simulink model "sensorFusionWithControlTB66"  (R2024a)
settings: Solver=FixedStepAuto  StartTime=0.0  StopTime=inf  FixedStep=controlRate  RelTol=1e-3
InitFcn:
  | modelParamsDD = Simulink.data.dictionary.open('modelConfigData.sldd');
  | sectModel = getSection(modelParamsDD,'Design Data');
  | controlRateTemp = getValue(getEntry(sectModel,'controlRate'));
  | 
  | measRate = controlRateTemp;
  | angleEstRate = measRate;
  | stateEstRate = measRate;
  | 
  | % Complementary filter
  | fc = 5; %Hz
  | tau = 1/(2*pi*fc);
  | % alpha = tau/(tau+controlRateTemp);
  | alpha = 0.98;
  | 
  | % Control params
  | tiltSetPoint = 5; % degree
  | D_min = 0;
  | 
  | % Tilt angle PID
  | Tw = 1;
  | Kp = 28;
  | Ki = 10; % At 100 Hz
  | Kd = 0;
  | 
  | 
  | clear controlRateTemp
undefined symbols (not defined in the file or in its folder): accelToUnit, controlRate, gyroToUnit, MaxMotorVoltage
libraries: stm32f7xxblockslib x2, stm32f4xxblockslib x1
settings Model: DataDictionary=globalData.sldd  VariantConfigurationObject=RobotVariantConfig  STM32="{\"PWMOutput\":[{\"ID\":\"sensorFusionWithControlTB66:205\"},{\"ID\":\"sensorFusionWithControlTB66:189\"}],\"DigitalPortWrite\":[{\"ID\":\"sensorFusionWithControlTB66:1189\"},{\"ID\":\"sensorFusionWithControlTB66:1220\"},{\"ID\":\"sensorFusionWithControlTB66:1221\"},{\"ID\":\"sensorFusionWithControlTB66:1222\"},{\"ID\":\"sensorFusionWithControlTB66:1223\"},{\"ID\":\"sensorFusionWithControlTB66:1225:7\"},{\"ID\":\"sensorFusionWithControlTB66:1225:8\"},{\"ID\":\"sensorFusionWithControlTB66:1225:9\"},{\"ID\":\"sensorFusionWithControlTB66:1225:10\"}],\"I2CControllerRead\":[{\"ID\":\"sensorFusionWithControlTB66:1237:7\"},{\"ID\":\"sensorFusionWithControlTB66:1237:18\"},{\"ID\":\"sensorFusionWithControlTB66:1237:19\"},{\"ID\":\"sensorFusionWithControlTB66:1237:20\"},{\"ID\":\"sensorFusionWithControlTB66:1238:7\"},{\"ID\":\"sensorFusionWithControlTB66:1238:15\"},{\"ID\":\"sensorFusionWithControlTB66:1238:16\"},{\"ID\":\"sensorFusionWithControlTB66:1238:17\"}],\"I2CControllerWrite\":[{\"ID\":\"sensorFusionWithControlTB66:1237:21\"},{\"ID\":\"sensorFusionWithControlTB66:1237:22\"},{\"ID\":\"sensorFusionWithControlTB66:1237:23\"},{\"ID\":\"sensorFusionWithControlTB66:1238:18\"},{\"ID\":\"sensorFusionWithControlTB66:1238:19\"},{\"ID\":\"sensorFusionWithControlTB66:1238:20\"}]}"  SimulationMode=external  Creator=Peter  LastModifiedBy=Peter
settings OptimizationCC: OptimizeBlockIOStorage=off  BufferReuse=off  ReuseModelBlockBuffer=off  GlobalBufferReuse=off  ExpressionFolding=off  EnableMemcpy=off  PassReuseOutputArgsAs=Individual arguments  LocalBlockOutputs=off  ZeroExternalMemoryAtStartup=off  ZeroInternalMemoryAtStartup=off  MaxStackSize=64  OptimizeDataStoreBuffers=off  BusAssignmentInplaceUpdate=off  OptimizationLevel=level0  OptimizationCustomize=off  EfficientTunableParamExpr=on
settings DebuggingCC: ParameterTunabilityLossMsg=error
settings HardwareCC: ProdBitPerPointer=32  ProdBitPerSizeT=32  ProdBitPerPtrDiffT=32  ProdLargestAtomicInteger=Long  ProdLargestAtomicFloat=Double  ProdWordSize=32  ProdLongLongMode=on  ProdHWDeviceType=ARM Compatible->ARM Cortex-M
settings SFSimCC: MATLABDynamicMemAlloc=off
settings RTWCC: Description=Embedded Coder  SystemTargetFile=ert.tlc  HardwareBoard=STM32F7xx Based (Single precision FPU)  TemplateMakefile=ert_default_tmf  Toolchain=GNU Tools for ARM Embedded Processors
settings CodeAppCC: GenerateComments=off  IgnoreCustomStorageClasses=off  OperatorAnnotations=on  SimulinkDataObjDesc=on  SFDataObjDesc=on  SimulinkBlockComments=off
settings ERTTargetCC: TargetLangStandard=C99 (ISO)  CodeReplacementLibrary=ARM Cortex-M  SupportComplex=off  ExtMode=on  ExtModeTransport=3  ExtModeStaticAlloc=on  ExtModeStaticAllocSize=2048  ExtModeMexFile=ext_xcp  ExtModeMexArgs=1 'COM11' 115200  ExtModeIntrfLevel=Level2 - Open

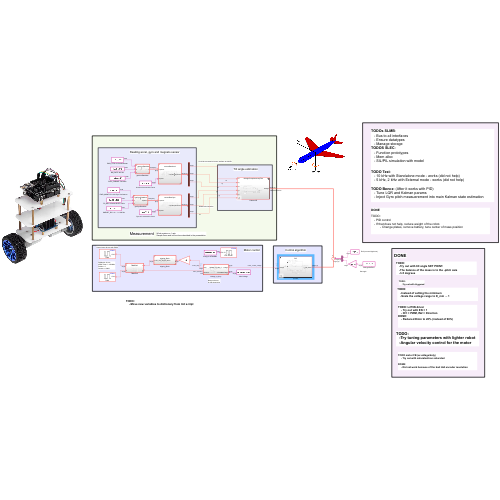
[thumbnail: Simulink's stored preview of the top-level diagram]
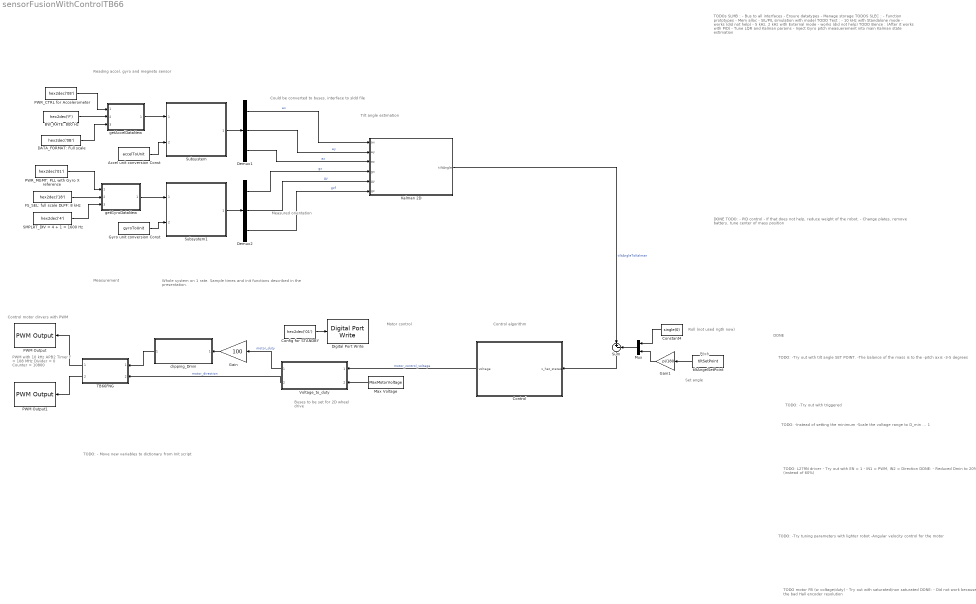
== system sensorFusionWithControlTB66 ==
  note: DONE
      |
      | TODO:
      | - PID control
      | - If that does not help, reduce weight of the robot.
      | - Change plates, remove battery, tune center of mass position
  note: TODO motor FB (w voltage/duty)
      | - Try out with saturated/non saturated
      |
      | DONE:
      | - Did not work because of the bad Hall encoder resolution
  note: TODO:
      | - Move new variables to dictionary from Init script
  note: TODO:
      | -Try tuning parameters with lighter robot
      | -Angular velocity control for the motor
  note: DONE
  note: TODO:
      | -Try out with triggered
  note: Pitch
  note: Roll (not used rigth now)
  note: Set angle
  note: TODO:
      | -Try out with tilt angle SET POINT.
      | -The balance of the mass is to the -pitch axis
      | -3-5 degrees
  note: Measured orientation
  note: TODOs SLMB :
      | - Bus to all interfaces
      | - Ensure datatypes
      | - Manage storage
      | TODOS SLEC :
      | - Function prototypes
      | - Mem alloc
      | - SIL/PIL simulation with model
      |
      | TODO Test :
      | - 10 kHz with Standalone mode - works (did not help)
      | - 5 kHz, 2 kHz with External mode - works (did not help)
      |
      | TODO Bence : (After it works with PID)
      | - Tune LQR and Kalman params
      | - Inject Gyro pitch measuerement into main Kalman state estimation
  note: PWM with 10 kHz
      | APB2 Timer f = 108 MHz
      | Divider = 0
      | Counter = 10800
  note: Whole system on 1 rate.
      | Sample times and init functions described in the presentation.
  note: Measurement
  note: Motor control
  note: Tilt angle estimation
  note: Buses to be set
      | for 2D wheel drive
  note: Control motor dirvers with PWM
  note: Could be converted to buses, interface to sldd file
  note: Reading accel, gyro and megneto sensor
  note: Control algorithm
  note: TODO:
      | -Instead of setting the minimum
      | -Scale the voltage range to D_min ... 1
  note: TODO: L279N driver
      | - Try out with EN = 1
      | - IN1 = PWM, IN2 = Direction
      | DONE:
      | - Reduced Dmin to 20% (instead of 60%)
  Accel unit conversion Const : Constant  Value=accelToUnit  OutDataTypeStr=single
  BW_RATE: 800 Hz : Constant  Value=hex2dec('F')  OutDataTypeStr=uint8
  Config for STANDBY : Constant  Value=hex2dec('01')  OutDataTypeStr=uint8
  Constant4 : Constant  Value=single(0)
  Control : Subsystem  Variant=on  VariantChoicesEnumeration=controlEnum  VariantControlVariable=controlAlgCtrl  VariantControl=Subsystem2  VariantActivationTime=inherit from Simulink.VariantControl
  DATA_FORMAT: Full scale : Constant  Value=hex2dec('0B')  OutDataTypeStr=uint8
  Demux1 : Demux  Outputs=3
  Demux2 : Demux  Outputs=3
  Digital Port Write : stm32f4xxblockslib/Digital Port Write  PortName=GPIOF  PinNumber=[13]  ReadOperation=off  IOAsArray=off  EnableSimPort=off  hoistedMaskSrc=ECSoC/ECSimCodegen/Digital Port Write
      settings: LibrarySourceBlock=stm32f7xxblockslib/Digital Port Write
  FS_SEL: full scale DLPF: 8 kHz : Constant  Value=hex2dec('18')  OutDataTypeStr=uint8
  Gain : Gain  Gain=100  OutDataTypeStr=single
  Gain1 : Gain  Gain=pi/180  ParamDataTypeStr=single
  Gyro unit conversion Const : Constant  Value=gyroToUnit  OutDataTypeStr=single
  Kalman 2D : Subsystem  Variant=on  VariantChoicesEnumeration=tiltEnum  VariantControlVariable=tiltEstCtrl  VariantControl=Kalman 2D  VariantActivationTime=inherit from Simulink.VariantControl
  Max Voltage : Constant  Value=MaxMotorVoltage  OutDataTypeStr=single
  Mux : Mux  Inputs=2
  PWM Output : stm32f7xxblockslib/PWM Output  TimerModule=TIM8  DutycycleUnits=Percentage  EnableChannel1=off  EnableChannel2=off  EnableChannel3=on  EnableChannel4=off  EnableChannel5=off  EnableChannel6=off  EnableCounterInput=off  EnableMainOutputInput=off  EnableFrequencyInput=off  SetRCAfterCE=off  OutputDirection=off  OutputMainOutputEnableStatus=off  SampleTime=0.1  EnableSimPort=off  EnableUpdateEvent=off  EnableCaptureCompare1Event=off  EnableCaptureCompare2Event=off  EnableCaptureCompare3Event=off  EnableCaptureCompare4Event=off  EnableTriggerEvent=off  EnableBreakEvent=off  EnableBreakEvent2=off  ProcessorFamily=STM32F7  hoistedMaskSrc=ECSoC/ECSimCodegen/PWM Output
  PWM Output1 : stm32f7xxblockslib/PWM Output  TimerModule=TIM8  DutycycleUnits=Percentage  EnableChannel1=off  EnableChannel2=off  EnableChannel3=off  EnableChannel4=on  EnableChannel5=off  EnableChannel6=off  EnableCounterInput=off  EnableMainOutputInput=off  EnableFrequencyInput=off  SetRCAfterCE=off  OutputDirection=off  OutputMainOutputEnableStatus=off  SampleTime=0.1  EnableSimPort=off  EnableUpdateEvent=off  EnableCaptureCompare1Event=off  EnableCaptureCompare2Event=off  EnableCaptureCompare3Event=off  EnableCaptureCompare4Event=off  EnableTriggerEvent=off  EnableBreakEvent=off  EnableBreakEvent2=off  ProcessorFamily=STM32F7  hoistedMaskSrc=ECSoC/ECSimCodegen/PWM Output
  PWR_CTRL for Accelerometer : Constant  Value=hex2dec('08')  OutDataTypeStr=uint8
  PWR_MGMT: PLL with Gyro X reference : Constant  Value=hex2dec('01')  OutDataTypeStr=uint8
  SMPLRT_DIV = 4 + 1 = 1600 Hz : Constant  Value=hex2dec('4')  OutDataTypeStr=uint8
  Subsystem : Subsystem  TreatAsAtomicUnit=on  SystemSampleTime=angleEstRate  ReferencedSubsystem=convertRawAccel
  Subsystem1 : Subsystem  TreatAsAtomicUnit=on  SystemSampleTime=angleEstRate  ReferencedSubsystem=convertRawGyro
  Sum : Sum  Inputs=|+-
  TB66FNG : Subsystem  TreatAsAtomicUnit=on  SystemSampleTime=controlRate  ReferencedSubsystem=TB66FNG
  Voltage_to_duty : Subsystem  TreatAsAtomicUnit=on  SystemSampleTime=controlRate  ReferencedSubsystem=Voltage_to_duty_1
  clipping_Dmin : Subsystem  TreatAsAtomicUnit=on  SystemSampleTime=controlRate  ReferencedSubsystem=clipping_Dmin
  getAccelDataNew : Subsystem  TreatAsAtomicUnit=on  ReferencedSubsystem=getAccelDataNew
  getGyroDataNew : Subsystem  TreatAsAtomicUnit=on  ReferencedSubsystem=getGyroDataNew
  tiltAngelSetPoint : Constant  Value=tiltSetPoint  OutDataTypeStr=single
  wires:
  Max Voltage/1 -> Voltage_to_duty/2
  Gyro unit conversion Const/1 -> Subsystem1/2
  Subsystem1/1 -> Demux2/1
  PWR_MGMT: PLL with Gyro X reference/1 -> getGyroDataNew/1
  getGyroDataNew/1 -> Subsystem1/1
  Kalman 2D/1(tiltAngle) -> Sum/1  "tiltAngleToKalman"
  Demux1/1 -> Kalman 2D/1(ax)  "ax"
  Demux1/2 -> Kalman 2D/2(ay)  "ay"
  Demux1/3 -> Kalman 2D/3(az)  "az"
  Demux2/3 -> Kalman 2D/6(gz)  "gzf"
  getAccelDataNew/1 -> Subsystem/1
  Accel unit conversion Const/1 -> Subsystem/2
  Subsystem/1 -> Demux1/1
  Control/1(voltage) -> Voltage_to_duty/1  "motor_control_voltage"
  Demux2/1 -> Kalman 2D/4(gx)  "gx"
  Demux2/2 -> Kalman 2D/5(gy)  "gy"
  BW_RATE: 800 Hz/1 -> getAccelDataNew/2
  PWR_CTRL for Accelerometer/1 -> getAccelDataNew/1
  FS_SEL: full scale DLPF: 8 kHz/1 -> getGyroDataNew/2
  SMPLRT_DIV = 4 + 1 = 1600 Hz/1 -> getGyroDataNew/3
  Sum/1 -> Control/1(x_hat_states)
  Mux/1 -> Sum/2
  Constant4/1 -> Mux/1
  tiltAngelSetPoint/1 -> Gain1/1
  Voltage_to_duty/1 -> Gain/1  "motor_duty"
  Voltage_to_duty/2 -> TB66FNG/2  "motor_direction"
  TB66FNG/1 -> PWM Output/1
  TB66FNG/2 -> PWM Output1/1
  clipping_Dmin/1 -> TB66FNG/1
  Gain/1 -> clipping_Dmin/1
  Config for STANDBY/1 -> Digital Port Write/1
  DATA_FORMAT: Full scale/1 -> getAccelDataNew/3
  Gain1/1 -> Mux/2

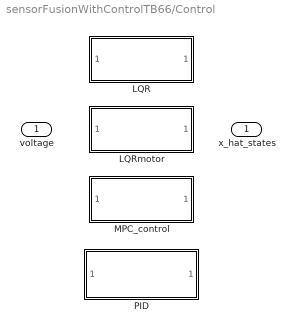
== system sensorFusionWithControlTB66/Control ==
  x_hat_states : Inport  OutDataTypeStr=single
  LQR : Subsystem  TreatAsAtomicUnit=on  SystemSampleTime=controlRate  VariantControl=controlAlgCtrl == controlEnum.LQR  ReferencedSubsystem=LQR
  LQRmotor : Subsystem  TreatAsAtomicUnit=on  SystemSampleTime=controlRate  VariantControl=controlAlgCtrl == controlEnum.LQRmotor  ReferencedSubsystem=LQRmotor
  MPC_control : Subsystem  TreatAsAtomicUnit=on  SystemSampleTime=controlRate  VariantControl=controlAlgCtrl == controlEnum.MPC_control  ReferencedSubsystem=MPC_control
  PID : Subsystem  VariantControl=controlAlgCtrl == controlEnum.PID  ReferencedSubsystem=PID
  voltage : Outport  OutDataTypeStr=single

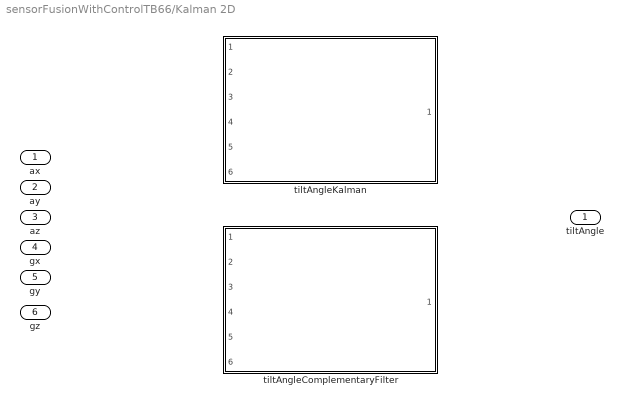
== system sensorFusionWithControlTB66/Kalman 2D ==
  ax : Inport
  ay : Inport  Port=2
  az : Inport  Port=3
  gx : Inport  Port=4
  gy : Inport  Port=5
  gz : Inport  Port=6
  tiltAngleComplementaryFilter : Subsystem  TreatAsAtomicUnit=on  SystemSampleTime=controlRate  VariantControl=tiltEstCtrl == tiltEnum.tiltAngleComplementaryFilter  ReferencedSubsystem=tiltAngleComplementaryFilter
  tiltAngleKalman : Subsystem  TreatAsAtomicUnit=on  SystemSampleTime=angleEstRate  VariantControl=tiltEstCtrl == tiltEnum.tiltAngleKalman  ReferencedSubsystem=tiltAngleKalman
  tiltAngle : Outport
